simulink model "circuit"  (R2015a)
settings: Solver=ode4  StartTime=0.0  StopTime=10  FixedStep=0.0001  RelTol=1e-3
settings Model: Creator=Aranya Dan  LastModifiedBy=Aranya Dan

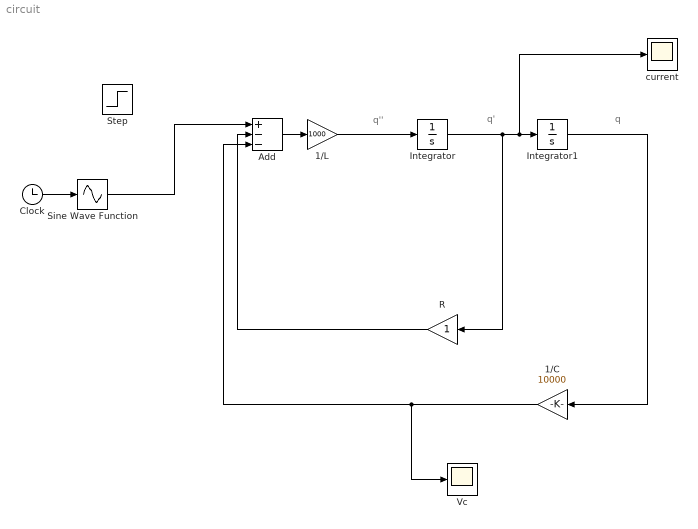
== system circuit ==
  note: q
  note: q'
  note: q''
  1/C : Gain  Gain=10000
  1/L : Gain  Gain=1000
  Add : Sum  Inputs=+--
  Clock : Clock
  Integrator : Integrator
  Integrator1 : Integrator
  R : Gain
  Sine Wave Function : Sin  TimeSource=Use external signal  SampleTime=0
  Step : Step  Time=0  After=10  SampleTime=0
  Vc : Scope
  current : Scope
  wires:
  Integrator/1 -> R/1, current/1, Integrator1/1
  Integrator1/1 -> 1/C/1
  1/L/1 -> Integrator/1
  Add/1 -> 1/L/1
  R/1 -> Add/2
  1/C/1 -> Vc/1, Add/3
  Sine Wave Function/1 -> Add/1
  Clock/1 -> Sine Wave Function/1
